simulink model "chap9_2sim"  (Simulink 8.1)
settings: Solver=ode45  StartTime=0.0  StopTime=30  FixedStep=0.005  RelTol=1e-3
settings Model: Creator=hp  LastModifiedBy=liujk  ExtModeTrigMode=oneshot  ExtModeArmWhenConnect=off
settings DataIOCC: LimitDataPoints=off  SignalLoggingName=sigsOut
settings OptimizationCC: BooleanDataType=off  InitFltsAndDblsToZero=on
settings DebuggingCC: SaveWithParameterizedLinksMsg=none  SignalResolutionControl=TryResolveAllWithWarning  SolverPrmCheckMsg=none  MultiTaskDSMMsg=warning  MultiTaskCondExecSysMsg=none  StrictBusMsg=None
settings HardwareCC: TargetUnknown=on
settings RTWCC: IncludeERTFirstTime=on
settings GRTTargetCC: TargetFcnLib=ansi_tfl_tmw.mat

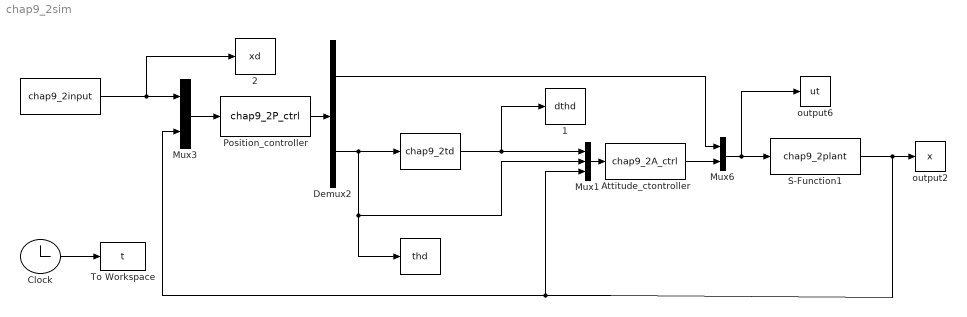
== system chap9_2sim ==
  " " : S-Function  FunctionName=chap9_2input  EnableBusSupport=off
  "  " : S-Function  FunctionName=chap9_2td  EnableBusSupport=off
  "   " : ToWorkspace  VariableName=thd  SampleTime=-1
  "   1" : ToWorkspace  VariableName=dthd  SampleTime=-1
  "   2" : ToWorkspace  VariableName=xd  SampleTime=-1
  Attitude_ctontroller : S-Function  FunctionName=chap9_2A_ctrl  EnableBusSupport=off
  Clock : Clock
  Demux2 : Demux  Outputs=2
  Mux1 : Mux  Inputs=3
  Mux3 : Mux  Inputs=2
  Mux6 : Mux  Inputs=2
  Position_controller : S-Function  FunctionName=chap9_2P_ctrl  EnableBusSupport=off
  S-Function1 : S-Function  FunctionName=chap9_2plant  EnableBusSupport=off
  To Workspace : ToWorkspace  VariableName=t  SampleTime=-1
  output2 : ToWorkspace  VariableName=x  SampleTime=-1
  output6 : ToWorkspace  VariableName=ut  SampleTime=-1
  wires:
  Clock/1 -> To Workspace/1
  Demux2/1 -> Mux6/1
  Mux1/1 -> Attitude_ctontroller/1
  Position_controller/1 -> Demux2/1
  Mux6/1 -> S-Function1/1, output6/1
  S-Function1/1 -> output2/1, Mux3/2, Mux1/3
  " "/1 -> "   2"/1, Mux3/1
  Mux3/1 -> Position_controller/1
  Attitude_ctontroller/1 -> Mux6/2
  "  "/1 -> "   1"/1, Mux1/1
  Demux2/2 -> "   "/1, Mux1/2, "  "/1
